simulink model "linearnilqr"  (R2020b)
settings: Solver=VariableStepAuto  StartTime=0.0  StopTime=10.0  RelTol=1e-3
values from neighbouring files (symbols this model uses):
  b1 = 0.0050134512    [I_PD.m]    (also in LQR.m = 0.05; PODACI.m = 0.05; Untitled2.m)
  b2 = 45    [LQR.m]    (also in PODACI.m)
  c = 0.03    [LQR.m]    (also in PODACI.m)
  d = 0.062    [LQR.m]    (also in PODACI.m)
  g = 9.81    [LQR.m]    (also in PODACI.m)
  K = lqr(A,B,Q,R)    [LQR.m]
  M = 1.2    [LQR.m]    (also in PODACI.m)
  m = 0.3    [LQR.m]    (also in PODACI.m)
settings Model: Creator=Toni  LastModifiedBy=Toni

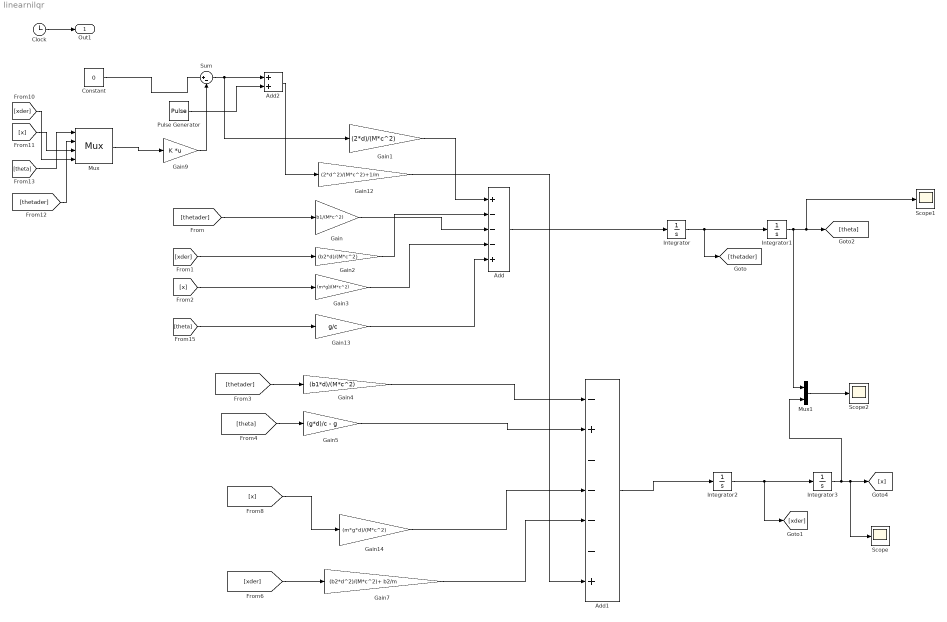
== system linearnilqr ==
  Add : Sum  Inputs=+---+
  Add1 : Sum  Inputs=-+----+
  Add2 : Sum
  Clock : Clock
  Constant : Constant  Value=0
  Gain : Gain  Gain=b1/(M*c^2)
  Gain1 : Gain  Gain=(2*d)/(M*c^2)
  Gain12 : Gain  Gain=(2*d^2)/(M*c^2)+1/m
  Gain13 : Gain  Gain=g/c
  Gain14 : Gain  Gain=(m*g*d)/(M*c^2)
  Gain2 : Gain  Gain=(b2*d)/(M*c^2)
  Gain3 : Gain  Gain=(m*g)/(M*c^2)
  Gain4 : Gain  Gain=(b1*d)/(M*c^2)
  Gain5 : Gain  Gain=(g*d)/c - g
  Gain7 : Gain  Gain=(b2*d^2)/(M*c^2)+ b2/m
  Gain9 : Gain  Gain=K  Multiplication=Matrix(K*u)
  Integrator{,1..3} (4 alike) : Integrator
  Mux : Mux
  Mux1 : Mux  Inputs=2
  Pulse Generator : DiscretePulseGenerator  PulseType=Time based  Period=10  PulseWidth=5
  Scope : Scope
  Scope1 : Scope
  Scope2 : Scope
  Sum : Sum  Inputs=|+-
  Out1 : Outport
  wires:
  Gain2/1 -> Add/2
  [xder] -> Gain7/1
  Gain/1 -> Add/3
  Gain14/1 -> Add1/4
  Gain5/1 -> Add1/2
  Add/1 -> Integrator/1
  Gain4/1 -> Add1/1
  [thetader] -> Gain4/1
  Gain12/1 -> Add1/7
  Integrator1/1 -> [theta], Scope1/1, Mux1/1
  Gain13/1 -> Add/5
  Integrator2/1 -> [xder], Integrator3/1
  [x] -> Gain3/1
  [thetader] -> Gain/1
  Integrator/1 -> Integrator1/1, [thetader]
  Add1/1 -> Integrator2/1
  [x] -> Gain14/1
  Gain7/1 -> Add1/5
  Gain3/1 -> Add/4
  Integrator3/1 -> Mux1/2, Scope/1, [x]
  [theta] -> Gain5/1
  [theta] -> Gain13/1
  [xder] -> Gain2/1
  Gain1/1 -> Add/1
  Mux/1 -> Gain9/1
  Clock/1 -> Out1/1
  Gain9/1 -> Sum/2
  [theta] -> Mux/1
  [thetader] -> Mux/2
  [x] -> Mux/3
  [xder] -> Mux/4
  Sum/1 -> Gain1/1, Add2/1
  Pulse Generator/1 -> Add2/2
  Add2/1 -> Gain12/1
  Mux1/1 -> Scope2/1
  Constant/1 -> ?
